simulink model "Simplus_1GFM_2OFF"  (R2022b)
settings: Solver=ode3  StartTime=0.0  StopTime=24  FixedStep=Ts  RelTol=1e-3  EnableMultiTasking=on
InitFcn:
  | Ts = 100e-6;
model workspace (MAT data in the model file):
  Fbase = 50
  Filter_Ind = 0.00435
  Shunt_C = 2.2e-06
  Test_Interval = 3
  Ts = 0.0001
  VDCref = 48
undefined symbols (not defined in the file): DiscIntNeverNeededParam
libraries: rtpi x45, spsabctodq0Lib x2, spsdq0toabcLib x1
settings Model: ModifiedByFormat=The MathWorks Inc.  SimulationMode=external  ExtModeTrigDuration=240000  ExtModeLogAll=off  Creator=The MathWorks, Inc.  LastModifiedBy=The MathWorks Inc.
settings SolverCC: AlgebraicLoopSolver=TrustRegion  PositivePriorityOrder=on  AutoInsertRateTranBlk=on
settings DataIOCC: LimitDataPoints=on  SaveFormat=Array  ReturnWorkspaceOutputs=off
settings OptimizationCC: EnhancedBackFolding=on  PassReuseOutputArgsThreshold=0  LocalBlockOutputs=off  EfficientMapNaN2IntZero=off  MaxStackSize=64  OptimizeBlockOrder=speed  DifferentSizesBufferReuse=on
settings DebuggingCC: UnderspecifiedInitializationDetection=Classic  MergeDetectMultiDrivingBlocksExec=none  SolverPrmCheckMsg=warning  ParameterTunabilityLossMsg=error  UnconnectedInputMsg=warning  UnconnectedOutputMsg=warning  UnconnectedLineMsg=warning  AllowSymbolicDim=off  SFUnexpectedBacktrackingDiag=warning  SFNoUnconditionalDefaultTransitionDiag=warning  SFExecutionAtInitializationDiag=none  SFMachineParentedDataDiag=warning  ArithmeticOperatorsInVariantConditions=warning
settings HardwareCC: ProdBitPerPointer=32  ProdBitPerSizeT=32  ProdBitPerPtrDiffT=32  ProdLargestAtomicInteger=Long  ProdLargestAtomicFloat=Double  ProdWordSize=32  ProdHWDeviceType=ARM Compatible->ARM Cortex  UseEmbeddedCoderFeatures=off
settings ModelReferenceCC: EnableRefExpFcnMdlSchedulingChecks=on  PropagateSignalLabelsOutOfModel=off
settings SFSimCC: SimUseLocalCustomCode=off  SimParseCustomCode=off  MATLABDynamicMemAlloc=off  CustomCodeUndefinedFunction=UseInterfaceOnly
settings RTWCC: Description=Simplus  SystemTargetFile=simplus.tlc  TemplateMakefile=simplex.tmf  RTWUseLocalCustomCode=off  RTWUseSimCustomCode=on  Toolchain=Simplus Xenomai ARM32  BuildConfiguration=Faster Runs
settings CodeAppCC: OperatorAnnotations=on  MangleLength=10  StateflowObjectComments=on
settings STFCustomTargetCC: TargetLangStandard=C99 (ISO)  GenerateFullHeader=off  ConcurrentExecutionCompliant=on  GRTInterface=on  UseToolchainInfoCompliant=on  SystemTargetFile=simplus.tlc
settings GRTTargetCC: GenerateFullHeader=off  ParMdlRefBuildCompliant=off  CompOptLevelCompliant=off  CombineOutputUpdateFcns=off  MatFileLogging=off  CPPClassGenCompliant=off  GRTInterface=on  ExtMode=on  ExtModeMexArgs='192.168.10.109', 0, 17725
settings ConfigComp: CovMetricSettings=dw  CovSaveCumulativeToWorkspaceVar=on  CovSaveSingleToWorkspaceVar=on  CovExternalEMLEnable=off  CovSFcnEnable=off

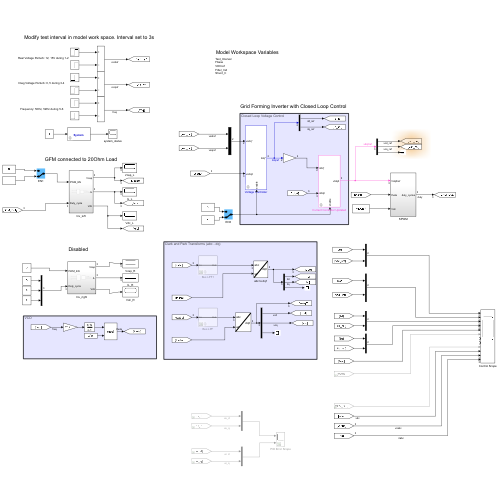
[thumbnail: Simulink's stored preview of the top-level diagram]
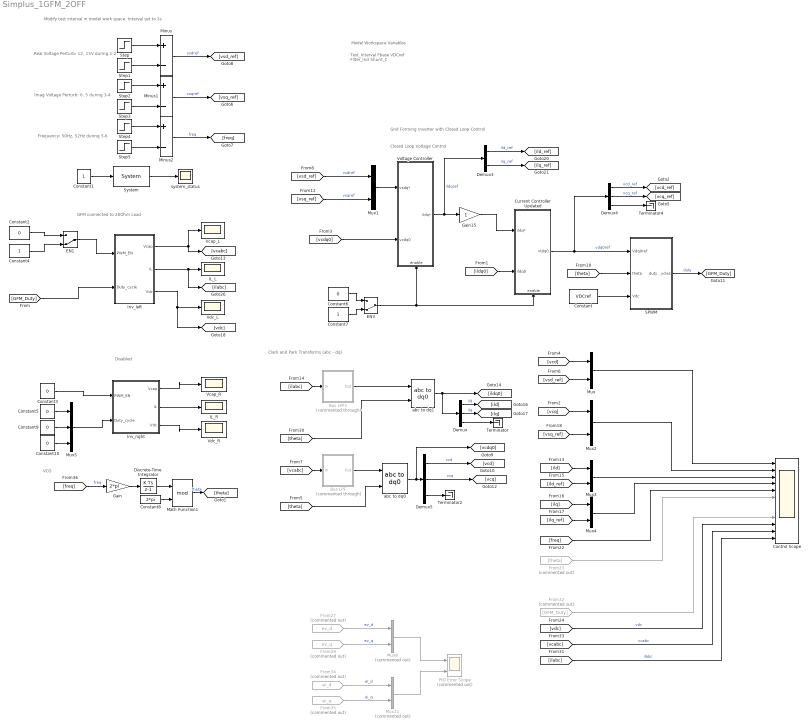
== system Simplus_1GFM_2OFF ==
  note: VCO
  note: Clark and Park Transforms (abc - dq)
  note: Closed Loop Voltage Control
  note: GFM connected to 20Ohm Load
  note: Test_Interval
      | Fbase
      | VDCref
      | Filter_Ind
      | Shunt_C
  note: Model Workspace Variables
  note: Disabled
  note: Grid Forming Inverter with Closed Loop Control
  note: Real Voltage Perturb: 12, 15V during 1-2
  note: Frequency: 50Hz, 52Hz during 5-6
  note: Imag Voltage Perturb: 0, 5 during 3-4
  note: Modify test interval in model work space. Interval set to 3s
  Bus LPF : Subsystem  Commented=through  mask{f_cutoff=1000}
      mask prompts: f_cutoff "Cutoff Frequency (Hz)"
      mask DialogControl Bus_LPF Prompt: Bus LPF
  Bus LPF1 : Subsystem  Commented=through  mask{f_cutoff=1000}
      mask prompts: f_cutoff "Cutoff Frequency (Hz)"
      mask DialogControl Bus_LPF Prompt: Bus LPF
  Constant : Constant  Value=VDCref
  Constant1 : Constant
  Constant{2..3,5..6,9..10} (6 alike) : Constant  Value=0
  Constant4 : Constant
  Constant7 : Constant
  Constant8 : Constant  Value=2*pi
  Control Scope : Scope  NumInputPorts=12
  Current Controller Updated : Subsystem  mask{Id_Proportional=0.61, Id_Integral=240}
      mask prompts: Id_Proportional "Kp"; Id_Integral "Ki"
      settings: PortSchema="{\"entries\":[{\"content\":{\"sides\":[{\"content\":{\"connectorIds\":[\"In1\",\"In2\"]},\"type\":\"ConnectorPlacement.EquallySpacedRectSide\",\"uuid\":\"134caf41-c34b-48d0-a71a-522329c40d8c\"},{\"content\":{\"connectorIds\":[\"Out1\"],\"side\":\"RIGHT\"},\"type\":\"ConnectorPlacement.EquallySpacedRectSide\",\"uuid\":\"de6d8359-09d9-4cb7-8990-bc4b6d48f18d\"},{\"content\":{\"connectorIds\":[],\"side\":\"TOP\"},\"type\":\"ConnectorPlacement.EquallySpacedRectSide\",\"uuid\":\"e2785d07-2ead-4d42-94ac-8025f550e46a\"},{\"content\":{\"connectorIds\":[\"In3\"],\"side\":\"BOTTOM\"},\"type\":\"ConnectorPlacement.EquallySpacedRectSide\",\"uuid\":\"a912a274-012c-4cba-911c-beb79bb7dc91\"}]},\"type\":\"ConnectorPlacement.EquallySpacedConnector\",\"uuid\":\"3c498838-bb9a-4b09-bf48-00f71cabf7b4\"}],\"packageUris\":[\"http://schema.mathworks.com/mf0/Connector/R2020b\"],\"version\":\"1.0\"}"
  Demux : Demux  Outputs=3
  Demux3 : Demux  Outputs=2
  Demux4 : Demux  Outputs=3
  Demux5 : Demux  Outputs=3
  Discrete-Time Integrator : DiscreteIntegrator  SampleTime=Ts  ICPrevOutput=DiscIntNeverNeededParam  ICPrevScaledInput=DiscIntNeverNeededParam
  EN1 : ManualSwitch  CurrentSetting=0
  EN3 : ManualSwitch  CurrentSetting=0
  From23 : From  Commented=on  GotoTag=theta
  From27 : From  Commented=on  GotoTag=ev_d  TagVisibility=global
      settings: CloseFcn=tagdialog Close
  From29 : From  Commented=on  GotoTag=ev_q  TagVisibility=global
      settings: CloseFcn=tagdialog Close
  From32 : From  Commented=on  GotoTag=GFM_Duty
      settings: CloseFcn=tagdialog Close
  From34 : From  Commented=on  GotoTag=ei_d
      settings: CloseFcn=tagdialog Close
  From35 : From  Commented=on  GotoTag=ei_q
      settings: CloseFcn=tagdialog Close
  Gain : Gain  Gain=2*pi
  Gain15 : Gain
  IL_L : Scope
  IL_R : Scope
  Inv_left : Subsystem
  Inv_right : Subsystem
  Math Function1 : Math  Operator=mod  SignedPower=on
  Minus : Sum  Inputs=+-
  Minus1 : Sum  Inputs=+-
  Minus2 : Sum  Inputs=+-
  Mux{,1..4} (5 alike) : Mux  Inputs=2
  Mux11 : Mux  Commented=on  Inputs=2
  Mux5 : Mux  Inputs=3
  Mux8 : Mux  Commented=on  Inputs=2
  PID Error Scope : Scope  Commented=on  NumInputPorts=2
  SPWM : Subsystem
  Step : Step  Time=Test_Interval*1  Before=12  After=15
  Step1 : Step  Time=Test_Interval*2  After=3
  Step2 : Step  Time=Test_Interval*3  After=5
  Step3 : Step  Time=Test_Interval*4  After=5
  Step4 : Step  Time=Test_Interval*5  Before=50  After=52  SampleTime=0
  Step5 : Step  Time=Test_Interval*6  After=2
  System : rtpi/System  Priority=-100  finger_print=015482637925  sync=Synchronous Series  div=4  estop=NONE
      settings: SourceProductName=Simplus Real-Time
  Terminator : Terminator
  Terminator2 : Terminator
  Terminator4 : Terminator
  Vcap_L : Scope
  Vcap_R : Scope
  Vdc_L : Scope
  Vdc_R : Scope
  Voltage Controller : Subsystem  mask{Id_Proportional=0.028, Id_Integral=8.685}
      mask prompts: Id_Proportional "Kp"; Id_Integral "Ki"
      settings: PortSchema="{\"entries\":[{\"content\":{\"sides\":[{\"content\":{\"connectorIds\":[\"In1\",\"In2\"]},\"type\":\"ConnectorPlacement.EquallySpacedRectSide\",\"uuid\":\"134caf41-c34b-48d0-a71a-522329c40d8c\"},{\"content\":{\"connectorIds\":[\"Out1\"],\"side\":\"RIGHT\"},\"type\":\"ConnectorPlacement.EquallySpacedRectSide\",\"uuid\":\"de6d8359-09d9-4cb7-8990-bc4b6d48f18d\"},{\"content\":{\"connectorIds\":[],\"side\":\"TOP\"},\"type\":\"ConnectorPlacement.EquallySpacedRectSide\",\"uuid\":\"e2785d07-2ead-4d42-94ac-8025f550e46a\"},{\"content\":{\"connectorIds\":[\"In3\"],\"side\":\"BOTTOM\"},\"type\":\"ConnectorPlacement.EquallySpacedRectSide\",\"uuid\":\"a912a274-012c-4cba-911c-beb79bb7dc91\"}]},\"type\":\"ConnectorPlacement.EquallySpacedConnector\",\"uuid\":\"3c498838-bb9a-4b09-bf48-00f71cabf7b4\"}],\"packageUris\":[\"http://schema.mathworks.com/mf0/Connector/R2020b\"],\"version\":\"1.0\"}"
  abc to dq0 : spsabctodq0Lib/abc to dq0  Alignment=90 degrees behind phase A axis
  abc to dq1 : spsabctodq0Lib/abc to dq0  Alignment=90 degrees behind phase A axis
  system_status : Scope
  wires:
  System/1 -> system_status/1
  Constant1/1 -> System/1
  Constant2/1 -> EN1/1
  Constant4/1 -> EN1/2
  EN1/1 -> Inv_left/1(PWM_EN)
  Inv_left/3(Vdc) -> [vdc], Vdc_L/1
  Inv_right/1(Vcap) -> Vcap_R/1
  Constant3/1 -> Inv_right/1(PWM_EN)
  Inv_right/2(IL) -> IL_R/1
  Demux4/2 -> [vcq_ref]  "vcq_ref"
  Demux/2 -> [ilq]  "ilq"
  Demux4/3 -> Terminator4/1
  Demux3/2 -> [ilq_ref]  "ilq_ref"
  Demux/3 -> Terminator/1
  Voltage Controller/1(ildq*) -> Gain15/1, Demux3/1  "ildqref"
  Current Controller Updated/1(vtdq0) -> Demux4/1, SPWM/1(Vdq0ref)  "vdq0ref"
  [theta] -> SPWM/2(theta)
  [ilabc] -> Bus LPF1/1(In)
  SPWM/1(duty_cycles) -> [GFM_Duty]  "duty"
  Demux/1 -> [ild]  "ild"
  EN3/1 -> Current Controller Updated/3(enable), Voltage Controller/3(enable)
  Demux3/1 -> [ild_ref]  "ild_ref"
  Demux4/1 -> [vcd_ref]  "vcd_ref"
  Constant/1 -> SPWM/3(Vdc)
  Gain15/1 -> Current Controller Updated/1(ildq*)
  Constant6/1 -> EN3/1
  Constant7/1 -> EN3/2
  [vcd] -> Mux/1
  [vcq] -> Mux2/1
  [ild] -> Mux3/1
  [ild_ref] -> Mux3/2
  [ilq] -> Mux4/1
  [ilq_ref] -> Mux4/2
  Mux/1 -> Control Scope/1
  Mux2/1 -> Control Scope/2
  Mux3/1 -> Control Scope/3
  Mux4/1 -> Control Scope/4
  From23/1 -> Control Scope/6
  Gain/1 -> Discrete-Time Integrator/1
  Discrete-Time Integrator/1 -> Math Function1/1
  Constant8/1 -> Math Function1/2
  [freq] -> Gain/1  "freq"
  Math Function1/1 -> [theta]  "theta"
  abc to dq0/1 -> [vcdq0], Demux5/1
  Demux5/1 -> [vcd]  "vcd"
  Demux5/3 -> Terminator2/1
  Demux5/2 -> [vcq]  "vcq"
  [vcabc] -> Bus LPF/1(In)
  [theta] -> abc to dq1/2
  abc to dq1/1 -> [ildq0], Demux/1
  [ilabc] -> Control Scope/12  "ilabc"
  [vcabc] -> Control Scope/11  "vcabc"
  From32/1 -> Control Scope/9
  [vcdq0] -> Voltage Controller/2(vcdq0)
  Bus LPF1/1(Out) -> abc to dq1/1
  [freq] -> Control Scope/5
  Inv_left/1(Vcap) -> Vcap_L/1, [vcabc]
  Inv_left/2(IL) -> [ilabc], IL_L/1
  [GFM_Duty] -> Inv_left/2(Duty_cycle)
  [vsq_ref] -> Mux1/2  "vsqref"
  Mux1/1 -> Voltage Controller/1(vsdq*)
  [vsd_ref] -> Mux1/1  "vsdref"
  Constant5/1 -> Mux5/1
  Constant9/1 -> Mux5/2
  Constant10/1 -> Mux5/3
  Mux5/1 -> Inv_right/2(Duty_cycle)
  [theta] -> abc to dq0/2
  [vsq_ref] -> Mux2/2
  [vsd_ref] -> Mux/2
  [vdc] -> Control Scope/10  "vdc"
  Inv_right/3(Vdc) -> Vdc_R/1
  Mux8/1 -> PID Error Scope/1
  From27/1 -> Mux8/1  "ev_d"
  From29/1 -> Mux8/2  "ev_q"
  From35/1 -> Mux11/2  "ei_q"
  Mux11/1 -> PID Error Scope/2
  From34/1 -> Mux11/1  "ei_d"
  Bus LPF/1(Out) -> abc to dq0/1
  [ildq0] -> Current Controller Updated/2(ildq0)
  Minus1/1 -> [vsq_ref]  "vsqref"
  Step3/1 -> Minus1/2
  Step5/1 -> Minus2/2
  Minus2/1 -> [freq]  "freq"
  Step4/1 -> Minus2/1
  Step2/1 -> Minus1/1
  Step/1 -> Minus/1
  Minus/1 -> [vsd_ref]  "vsdref"
  Step1/1 -> Minus/2

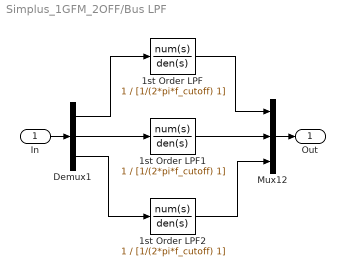
== system Simplus_1GFM_2OFF/Bus LPF ==
  In : Inport
  1st Order LPF : TransferFcn  Numerator=1  Denominator=[1/(2*pi*f_cutoff) 1]
  1st Order LPF1 : TransferFcn  Numerator=1  Denominator=[1/(2*pi*f_cutoff) 1]
  1st Order LPF2 : TransferFcn  Numerator=1  Denominator=[1/(2*pi*f_cutoff) 1]
  Demux1 : Demux  Outputs=3
  Mux12 : Mux  Inputs=3
  Out : Outport
  wires:
  Demux1/3 -> 1st Order LPF2/1
  Mux12/1 -> Out/1
  1st Order LPF/1 -> Mux12/1
  Demux1/1 -> 1st Order LPF/1
  Demux1/2 -> 1st Order LPF1/1
  1st Order LPF2/1 -> Mux12/3
  In/1 -> Demux1/1
  1st Order LPF1/1 -> Mux12/2

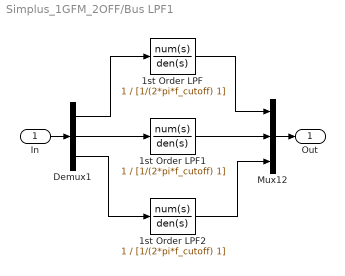
== system Simplus_1GFM_2OFF/Bus LPF1 ==
  In : Inport
  1st Order LPF : TransferFcn  Numerator=1  Denominator=[1/(2*pi*f_cutoff) 1]
  1st Order LPF1 : TransferFcn  Numerator=1  Denominator=[1/(2*pi*f_cutoff) 1]
  1st Order LPF2 : TransferFcn  Numerator=1  Denominator=[1/(2*pi*f_cutoff) 1]
  Demux1 : Demux  Outputs=3
  Mux12 : Mux  Inputs=3
  Out : Outport
  wires:
  Demux1/3 -> 1st Order LPF2/1
  Mux12/1 -> Out/1
  1st Order LPF/1 -> Mux12/1
  Demux1/1 -> 1st Order LPF/1
  Demux1/2 -> 1st Order LPF1/1
  1st Order LPF2/1 -> Mux12/3
  In/1 -> Demux1/1
  1st Order LPF1/1 -> Mux12/2

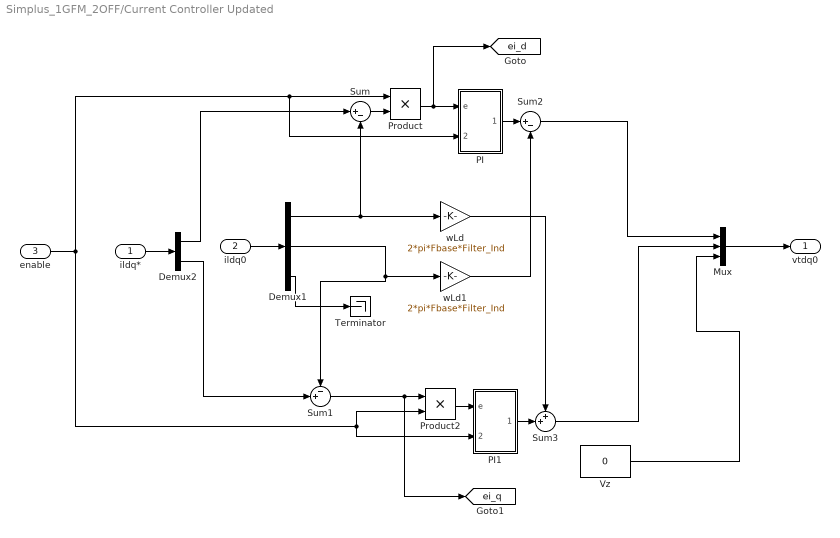
== system Simplus_1GFM_2OFF/Current Controller Updated ==
  ildq* : Inport
  ildq0 : Inport  Port=2
  enable : Inport  Port=3
  Demux1 : Demux  Outputs=3
  Demux2 : Demux  Outputs=2
  Mux : Mux  Inputs=3
  PI : Subsystem
  PI1 : Subsystem
  Product : Product  RndMeth=Zero
  Product2 : Product  RndMeth=Zero
  Sum : Sum  Inputs=|+-
  Sum1 : Sum  Inputs=-+|
  Sum2 : Sum  Inputs=|+-
  Sum3 : Sum  Inputs=++|
  Terminator : Terminator
  Vz : Constant  Value=0
  wLd : Gain  Gain=2*pi*Fbase*Filter_Ind
  wLd1 : Gain  Gain=2*pi*Fbase*Filter_Ind
  vtdq0 : Outport
  tag scope: ei_d=global, ei_q=global
  wires:
  Sum2/1 -> Mux/1
  Sum3/1 -> Mux/2
  ildq0/1 -> Demux1/1
  Mux/1 -> vtdq0/1
  Demux1/3 -> Terminator/1
  ildq*/1 -> Demux2/1
  Demux2/1 -> Sum/1
  Demux2/2 -> Sum1/2
  PI/1(Out) -> Sum2/1
  wLd/1 -> Sum3/1
  wLd1/1 -> Sum2/2
  PI1/1(Out) -> Sum3/2
  Demux1/2 -> Sum1/1, wLd1/1
  Demux1/1 -> wLd/1, Sum/2
  Product2/1 -> PI1/1(e)
  Sum/1 -> Product/2
  enable/1 -> Product/1, PI/2(RST), PI1/2(RST), Product2/2
  Vz/1 -> Mux/3
  Sum1/1 -> [ei_q], Product2/1
  Product/1 -> [ei_d], PI/1(e)

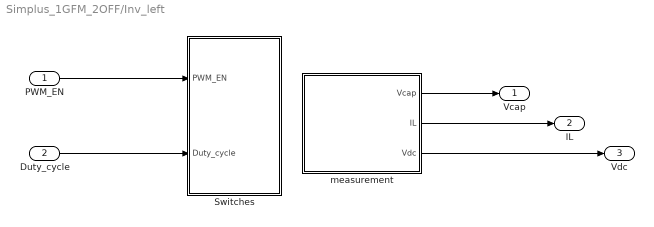
== system Simplus_1GFM_2OFF/Inv_left ==
  PWM_EN : Inport
  Duty_cycle : Inport  Port=2
  Switches : Subsystem
  measurement : Subsystem
  Vcap : Outport
  IL : Outport  Port=2
  Vdc : Outport  Port=3
  wires:
  Duty_cycle/1 -> Switches/2(Duty_cycle)
  PWM_EN/1 -> Switches/1(PWM_EN)
  measurement/3(Vdc) -> Vdc/1
  measurement/2(IL) -> IL/1
  measurement/1(Vcap) -> Vcap/1

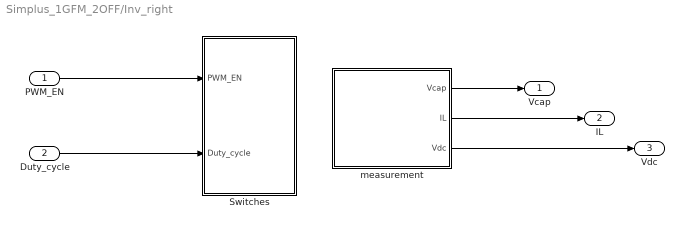
== system Simplus_1GFM_2OFF/Inv_right ==
  PWM_EN : Inport
  Duty_cycle : Inport  Port=2
  Switches : Subsystem
  measurement : Subsystem
  Vcap : Outport
  IL : Outport  Port=2
  Vdc : Outport  Port=3
  wires:
  measurement/1(Vcap) -> Vcap/1
  measurement/2(IL) -> IL/1
  measurement/3(Vdc) -> Vdc/1
  PWM_EN/1 -> Switches/1(PWM_EN)
  Duty_cycle/1 -> Switches/2(Duty_cycle)

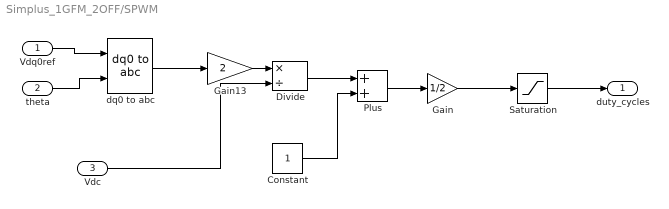
== system Simplus_1GFM_2OFF/SPWM ==
  Vdq0ref : Inport
  theta : Inport  Port=2
  Vdc : Inport  Port=3
  Constant : Constant
  Divide : Product  Inputs=*/
  Gain : Gain  Gain=1/2
  Gain13 : Gain  Gain=2
  Plus : Sum
  Saturation : Saturate  UpperLimit=0.9  LowerLimit=0.1
  dq0 to abc : spsdq0toabcLib/dq0 to abc  Alignment=90 degrees behind phase A axis
  duty_cycles : Outport
  wires:
  Vdq0ref/1 -> dq0 to abc/1
  Gain/1 -> Saturation/1
  theta/1 -> dq0 to abc/2
  Constant/1 -> Plus/2
  Plus/1 -> Gain/1
  Saturation/1 -> duty_cycles/1
  dq0 to abc/1 -> Gain13/1
  Gain13/1 -> Divide/1
  Vdc/1 -> Divide/2
  Divide/1 -> Plus/1

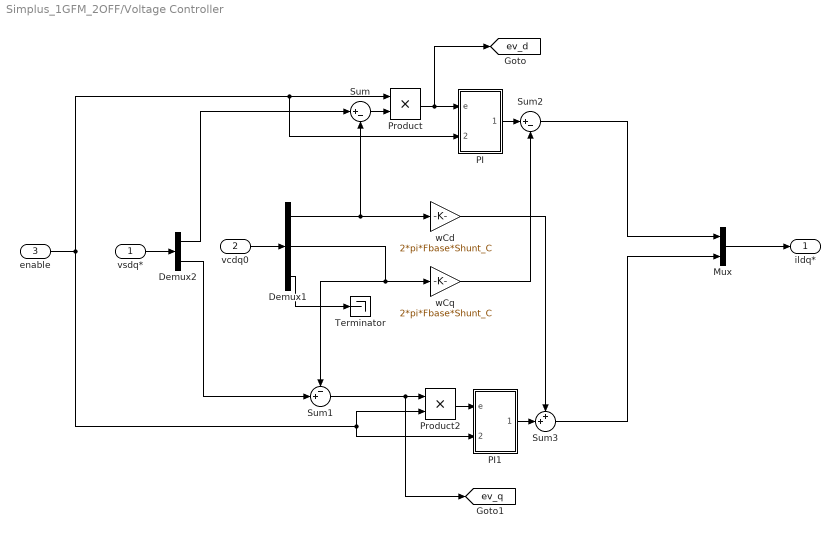
== system Simplus_1GFM_2OFF/Voltage Controller ==
  vsdq* : Inport
  vcdq0 : Inport  Port=2
  enable : Inport  Port=3
  Demux1 : Demux  Outputs=3
  Demux2 : Demux  Outputs=2
  Mux : Mux  Inputs=2
  PI : Subsystem
  PI1 : Subsystem
  Product : Product  RndMeth=Zero
  Product2 : Product  RndMeth=Zero
  Sum : Sum  Inputs=|+-
  Sum1 : Sum  Inputs=-+|
  Sum2 : Sum  Inputs=|+-
  Sum3 : Sum  Inputs=++|
  Terminator : Terminator
  wCd : Gain  Gain=2*pi*Fbase*Shunt_C
  wCq : Gain  Gain=2*pi*Fbase*Shunt_C
  ildq* : Outport
  tag scope: ev_d=global, ev_q=global
  wires:
  Sum2/1 -> Mux/1
  Sum3/1 -> Mux/2
  vcdq0/1 -> Demux1/1
  Mux/1 -> ildq*/1
  Demux1/3 -> Terminator/1
  vsdq*/1 -> Demux2/1
  Demux2/1 -> Sum/1
  Demux2/2 -> Sum1/2
  Product/1 -> [ev_d], PI/1(e)
  Sum1/1 -> [ev_q], Product2/1
  PI/1(Out) -> Sum2/1
  wCd/1 -> Sum3/1
  wCq/1 -> Sum2/2
  PI1/1(Out) -> Sum3/2
  Demux1/2 -> Sum1/1, wCq/1
  Demux1/1 -> wCd/1, Sum/2
  Product2/1 -> PI1/1(e)
  Sum/1 -> Product/2
  enable/1 -> Product/1, PI/2(RST), PI1/2(RST), Product2/2

== system Simplus_1GFM_2OFF/Current Controller Updated/PI ==
  e : Inport
  RST : Inport  Port=2
  Discrete-Time Integrator : DiscreteIntegrator  gainval=1  ExternalReset=either  SampleTime=Ts  LimitOutput=on  UpperSaturationLimit=20000  LowerSaturationLimit=-20000  ICPrevOutput=DiscIntNeverNeededParam  ICPrevScaledInput=DiscIntNeverNeededParam
  Ki : Gain  Gain=Id_Integral  SaturateOnIntegerOverflow=on  OutDataTypeStr=Inherit: Same as input  ParamDataTypeStr=Inherit: Same as input
  Kp : Gain  Gain=Id_Proportional  SaturateOnIntegerOverflow=on  OutDataTypeStr=Inherit: Same as input  ParamDataTypeStr=Inherit: Same as input
  Sum4 : Sum  SaturateOnIntegerOverflow=on
  Out : Outport
  wires:
  Ki/1 -> Discrete-Time Integrator/1
  Kp/1 -> Sum4/1
  e/1 -> Ki/1, Kp/1
  Discrete-Time Integrator/1 -> Sum4/2
  Sum4/1 -> Out/1
  RST/1 -> Discrete-Time Integrator/2

== system Simplus_1GFM_2OFF/Current Controller Updated/PI1 ==
  e : Inport
  RST : Inport  Port=2
  Discrete-Time Integrator : DiscreteIntegrator  gainval=1  ExternalReset=either  SampleTime=Ts  LimitOutput=on  UpperSaturationLimit=20000  LowerSaturationLimit=-20000  ICPrevOutput=DiscIntNeverNeededParam  ICPrevScaledInput=DiscIntNeverNeededParam
  Ki : Gain  Gain=Id_Integral  SaturateOnIntegerOverflow=on  OutDataTypeStr=Inherit: Same as input  ParamDataTypeStr=Inherit: Same as input
  Kp : Gain  Gain=Id_Proportional  SaturateOnIntegerOverflow=on  OutDataTypeStr=Inherit: Same as input  ParamDataTypeStr=Inherit: Same as input
  Sum4 : Sum  SaturateOnIntegerOverflow=on
  Out : Outport
  wires:
  Ki/1 -> Discrete-Time Integrator/1
  Kp/1 -> Sum4/1
  e/1 -> Ki/1, Kp/1
  Discrete-Time Integrator/1 -> Sum4/2
  Sum4/1 -> Out/1
  RST/1 -> Discrete-Time Integrator/2

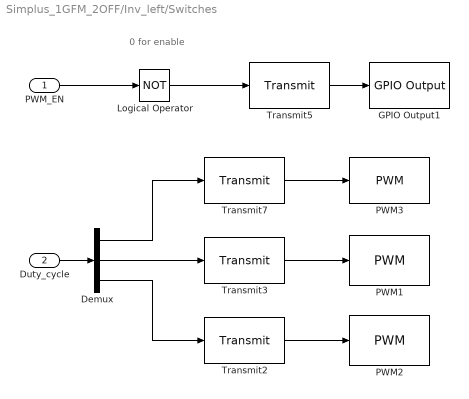
== system Simplus_1GFM_2OFF/Inv_left/Switches ==
  note: 0 for enable
  PWM_EN : Inport
  Duty_cycle : Inport  Port=2
  Demux : Demux  Outputs=3
  GPIO Output1 : rtpi/GPIO Output  finger_print=115482637925  blk_num=1  gpio_num=1  gpio1=18  od1=off  gpio2=0  od2=off  gpio3=0  od3=off  gpio4=0  od4=off  gpio5=0  od5=off  gpio6=0  od6=off  gpio7=0  od7=off  gpio8=0  od8=off  gpio9=0  od9=off  gpio10=0  od10=off  gpio11=0  od11=off  gpio12=0  od12=off  gpio13=0  od13=off  gpio14=0  od14=off  gpio15=0  od15=off  gpio16=0  od16=off  dir=1
      settings: SourceProductName=Simplus Real-Time
  Logical Operator : Logic  Operator=NOT  AllPortsSameDT=off  OutDataTypeStr=boolean
  PWM1 : rtpi/PWM  finger_print=115482637925  blk_num=1  pwmx=5  sync=on  mode=Normal  input=Duty Cycle  data_type=float  trigger_a=Zero  trigger_b=Zero  clock=1  tdead=2  period=10000  duty=0.5  phase=0.0
      settings: SourceProductName=Simplus Real-Time
  PWM2 : rtpi/PWM  finger_print=115482637925  blk_num=2  pwmx=6  sync=on  mode=Normal  input=Duty Cycle  data_type=float  trigger_a=Zero  trigger_b=Zero  clock=1  tdead=2  period=10000  duty=0.5  phase=0.0
      settings: SourceProductName=Simplus Real-Time
  PWM3 : rtpi/PWM  finger_print=115482637925  blk_num=3  pwmx=4  sync=on  mode=Normal  input=Duty Cycle  data_type=float  trigger_a=Zero  trigger_b=Zero  clock=1  tdead=2  period=10000  duty=0.5  phase=0.0
      settings: SourceProductName=Simplus Real-Time
  Transmit2 : rtpi/Transmit  Priority=10  finger_print=115482637925  blk_num=1  data_type=4  conv_type=single
      settings: SourceProductName=Simplus Real-Time
  Transmit3 : rtpi/Transmit  Priority=10  finger_print=115482637925  blk_num=2  data_type=4  conv_type=single
      settings: SourceProductName=Simplus Real-Time
  Transmit5 : rtpi/Transmit  finger_print=115482637925  blk_num=3  data_type=2  conv_type=uint16
      settings: SourceProductName=Simplus Real-Time
  Transmit7 : rtpi/Transmit  Priority=10  finger_print=115482637925  blk_num=4  data_type=4  conv_type=single
      settings: SourceProductName=Simplus Real-Time
  wires:
  Transmit2/1 -> PWM2/1
  Transmit3/1 -> PWM1/1
  Transmit7/1 -> PWM3/1
  Duty_cycle/1 -> Demux/1
  Demux/2 -> Transmit3/1
  Demux/1 -> Transmit7/1
  Demux/3 -> Transmit2/1
  Transmit5/1 -> GPIO Output1/1
  Logical Operator/1 -> Transmit5/1
  PWM_EN/1 -> Logical Operator/1

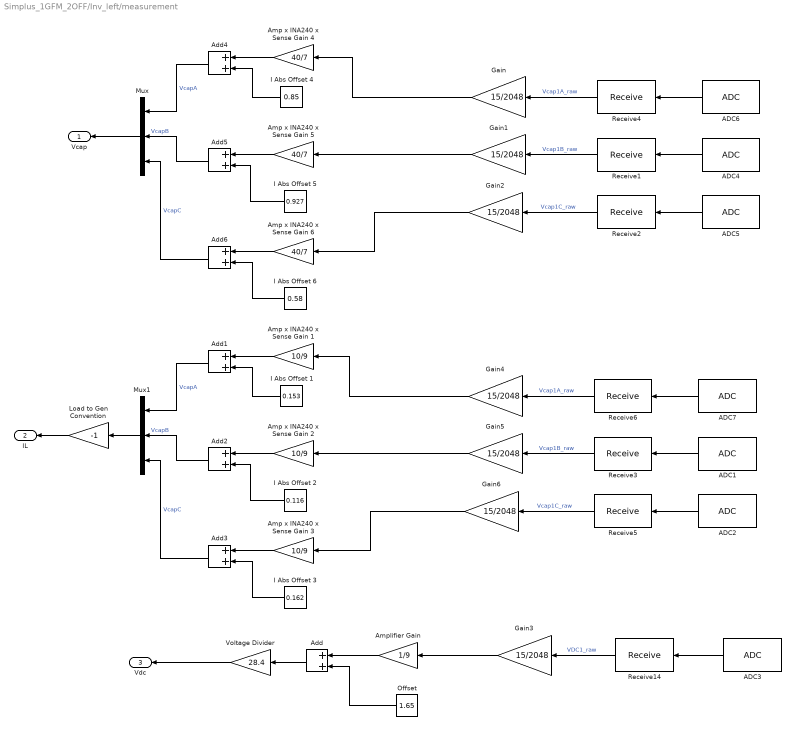
== system Simplus_1GFM_2OFF/Inv_left/measurement ==
  ADC1 : rtpi/ADC  finger_print=115482637925  blk_num=1  adcx=D  prior=2  pin=D2  trigger=PWM4A  data_type=int16  gain=1  rsrc=100  offset=AC  protect=Enabled  max=2000  min=-2000
      settings: SourceProductName=Simplus Real-Time
  ADC2 : rtpi/ADC  finger_print=115482637925  blk_num=2  adcx=D  prior=3  pin=D3  trigger=PWM4A  data_type=int16  gain=1  rsrc=100  offset=AC  protect=Enabled  max=2000  min=-2000
      settings: SourceProductName=Simplus Real-Time
  ADC3 : rtpi/ADC  finger_print=115482637925  blk_num=3  adcx=D  prior=4  pin=D4  trigger=PWM4A  data_type=int16  gain=1  rsrc=100  offset=AC  protect=Enabled  max=1500  min=-2048
      settings: SourceProductName=Simplus Real-Time
  ADC4 : rtpi/ADC  finger_print=115482637925  blk_num=4  adcx=C  prior=2  pin=C2  trigger=PWM4A  data_type=int16  gain=1  rsrc=100  offset=AC  protect=Enabled  max=2000  min=-2000
      settings: SourceProductName=Simplus Real-Time
  ADC5 : rtpi/ADC  finger_print=115482637925  blk_num=5  adcx=C  prior=3  pin=C3  trigger=PWM4A  data_type=int16  gain=1  rsrc=100  offset=AC  protect=Enabled  max=2000  min=-2000
      settings: SourceProductName=Simplus Real-Time
  ADC6 : rtpi/ADC  finger_print=115482637925  blk_num=6  adcx=C  prior=1  pin=C1  trigger=PWM4A  data_type=int16  gain=1  rsrc=100  offset=AC  protect=Enabled  max=2000  min=-2000
      settings: SourceProductName=Simplus Real-Time
  ADC7 : rtpi/ADC  finger_print=115482637925  blk_num=7  adcx=D  prior=1  pin=D1  trigger=PWM4A  data_type=int16  gain=1  rsrc=100  offset=AC  protect=Enabled  max=2000  min=-2000
      settings: SourceProductName=Simplus Real-Time
  Add{,1..6} (7 alike) : Sum
  Amp x INA240 x Sense Gain 1 : Gain  Gain=10/9
  Amp x INA240 x Sense Gain 2 : Gain  Gain=10/9
  Amp x INA240 x Sense Gain 3 : Gain  Gain=10/9
  Amp x INA240 x Sense Gain 4 : Gain  Gain=40/7
  Amp x INA240 x Sense Gain 5 : Gain  Gain=40/7
  Amp x INA240 x Sense Gain 6 : Gain  Gain=40/7
  Amplifier Gain : Gain  Gain=1/9
  Gain{,1..6} (7 alike) : Gain  Gain=15/2048
  I Abs Offset 1 : Constant  Value=0.153
  I Abs Offset 2 : Constant  Value=0.116
  I Abs Offset 3 : Constant  Value=0.162
  I Abs Offset 4 : Constant  Value=0.85
  I Abs Offset 5 : Constant  Value=0.927
  I Abs Offset 6 : Constant  Value=0.58
  Load to Gen Convention : Gain  Gain=-1
  Mux : Mux  Inputs=3
  Mux1 : Mux  Inputs=3
  Offset : Constant  Value=1.65
  Receive1 : rtpi/Receive  Priority=12  finger_print=115482637925  blk_num=1  data_type=2
      settings: SourceProductName=Simplus Real-Time
  Receive14 : rtpi/Receive  Priority=12  finger_print=115482637925  blk_num=2  data_type=2
      settings: SourceProductName=Simplus Real-Time
  Receive2 : rtpi/Receive  Priority=12  finger_print=115482637925  blk_num=3  data_type=2
      settings: SourceProductName=Simplus Real-Time
  Receive3 : rtpi/Receive  Priority=12  finger_print=115482637925  blk_num=4  data_type=2
      settings: SourceProductName=Simplus Real-Time
  Receive4 : rtpi/Receive  Priority=12  finger_print=115482637925  blk_num=5  data_type=2
      settings: SourceProductName=Simplus Real-Time
  Receive5 : rtpi/Receive  Priority=12  finger_print=115482637925  blk_num=6  data_type=2
      settings: SourceProductName=Simplus Real-Time
  Receive6 : rtpi/Receive  Priority=12  finger_print=115482637925  blk_num=7  data_type=2
      settings: SourceProductName=Simplus Real-Time
  Voltage Divider : Gain  Gain=28.4
  Vcap : Outport
  IL : Outport  Port=2
  Vdc : Outport  Port=3
  wires:
  ADC6/1 -> Receive4/1
  Receive4/1 -> Gain/1  "Vcap1A_raw"
  Amp x INA240 x Sense Gain 6/1 -> Add6/1
  I Abs Offset 6/1 -> Add6/2
  I Abs Offset 4/1 -> Add4/2
  Amp x INA240 x Sense Gain 4/1 -> Add4/1
  ADC5/1 -> Receive2/1
  Amp x INA240 x Sense Gain 5/1 -> Add5/1
  Receive1/1 -> Gain1/1  "Vcap1B_raw"
  I Abs Offset 5/1 -> Add5/2
  Receive2/1 -> Gain2/1  "Vcap1C_raw"
  ADC4/1 -> Receive1/1
  Amp x INA240 x Sense Gain 3/1 -> Add3/1
  Amp x INA240 x Sense Gain 1/1 -> Add1/1
  I Abs Offset 1/1 -> Add1/2
  Amp x INA240 x Sense Gain 2/1 -> Add2/1
  I Abs Offset 2/1 -> Add2/2
  I Abs Offset 3/1 -> Add3/2
  Receive14/1 -> Gain3/1  "VDC1_raw"
  ADC3/1 -> Receive14/1
  Add/1 -> Voltage Divider/1
  Amplifier Gain/1 -> Add/1
  Offset/1 -> Add/2
  Voltage Divider/1 -> Vdc/1
  Gain/1 -> Amp x INA240 x Sense Gain 4/1
  Gain1/1 -> Amp x INA240 x Sense Gain 5/1
  Gain2/1 -> Amp x INA240 x Sense Gain 6/1
  Gain3/1 -> Amplifier Gain/1
  Add4/1 -> Mux/1  "VcapA"
  Add5/1 -> Mux/2  "VcapB"
  Add6/1 -> Mux/3  "VcapC"
  Mux/1 -> Vcap/1
  ADC7/1 -> Receive6/1
  Gain4/1 -> Amp x INA240 x Sense Gain 1/1
  Gain5/1 -> Amp x INA240 x Sense Gain 2/1
  ADC1/1 -> Receive3/1
  ADC2/1 -> Receive5/1
  Receive3/1 -> Gain5/1  "Vcap1B_raw"
  Receive5/1 -> Gain6/1  "Vcap1C_raw"
  Gain6/1 -> Amp x INA240 x Sense Gain 3/1
  Receive6/1 -> Gain4/1  "Vcap1A_raw"
  Add3/1 -> Mux1/3  "VcapC"
  Mux1/1 -> Load to Gen Convention/1
  Add1/1 -> Mux1/1  "VcapA"
  Add2/1 -> Mux1/2  "VcapB"
  Load to Gen Convention/1 -> IL/1

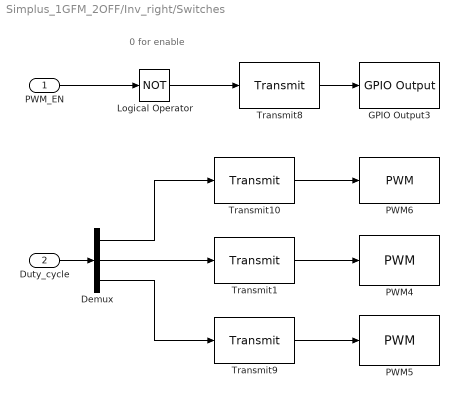
== system Simplus_1GFM_2OFF/Inv_right/Switches ==
  note: 0 for enable
  PWM_EN : Inport
  Duty_cycle : Inport  Port=2
  Demux : Demux  Outputs=3
  GPIO Output3 : rtpi/GPIO Output  finger_print=115482637925  blk_num=2  gpio_num=1  gpio1=24  od1=off  gpio2=0  od2=off  gpio3=0  od3=off  gpio4=0  od4=off  gpio5=0  od5=off  gpio6=0  od6=off  gpio7=0  od7=off  gpio8=0  od8=off  gpio9=0  od9=off  gpio10=0  od10=off  gpio11=0  od11=off  gpio12=0  od12=off  gpio13=0  od13=off  gpio14=0  od14=off  gpio15=0  od15=off  gpio16=0  od16=off  dir=1
      settings: SourceProductName=Simplus Real-Time
  Logical Operator : Logic  Operator=NOT  AllPortsSameDT=off  OutDataTypeStr=boolean
  PWM4 : rtpi/PWM  finger_print=115482637925  blk_num=4  pwmx=2  sync=on  mode=Normal  input=Duty Cycle  data_type=float  trigger_a=Zero  trigger_b=Zero  clock=1  tdead=2  period=10000  duty=0.5  phase=0.0
      settings: SourceProductName=Simplus Real-Time
  PWM5 : rtpi/PWM  finger_print=115482637925  blk_num=5  pwmx=3  sync=on  mode=Normal  input=Duty Cycle  data_type=float  trigger_a=Zero  trigger_b=Zero  clock=1  tdead=2  period=10000  duty=0.5  phase=0.0
      settings: SourceProductName=Simplus Real-Time
  PWM6 : rtpi/PWM  finger_print=115482637925  blk_num=6  pwmx=1  sync=on  mode=Normal  input=Duty Cycle  data_type=float  trigger_a=Zero  trigger_b=Zero  clock=1  tdead=2  period=10000  duty=0.5  phase=0.0
      settings: SourceProductName=Simplus Real-Time
  Transmit1 : rtpi/Transmit  Priority=10  finger_print=115482637925  blk_num=5  data_type=4  conv_type=single
      settings: SourceProductName=Simplus Real-Time
  Transmit10 : rtpi/Transmit  Priority=10  finger_print=115482637925  blk_num=6  data_type=4  conv_type=single
      settings: SourceProductName=Simplus Real-Time
  Transmit8 : rtpi/Transmit  finger_print=115482637925  blk_num=7  data_type=2  conv_type=uint16
      settings: SourceProductName=Simplus Real-Time
  Transmit9 : rtpi/Transmit  Priority=10  finger_print=115482637925  blk_num=8  data_type=4  conv_type=single
      settings: SourceProductName=Simplus Real-Time
  wires:
  Duty_cycle/1 -> Demux/1
  PWM_EN/1 -> Logical Operator/1
  Demux/3 -> Transmit9/1
  Demux/1 -> Transmit10/1
  Demux/2 -> Transmit1/1
  Transmit9/1 -> PWM5/1
  Transmit1/1 -> PWM4/1
  Transmit10/1 -> PWM6/1
  Transmit8/1 -> GPIO Output3/1
  Logical Operator/1 -> Transmit8/1

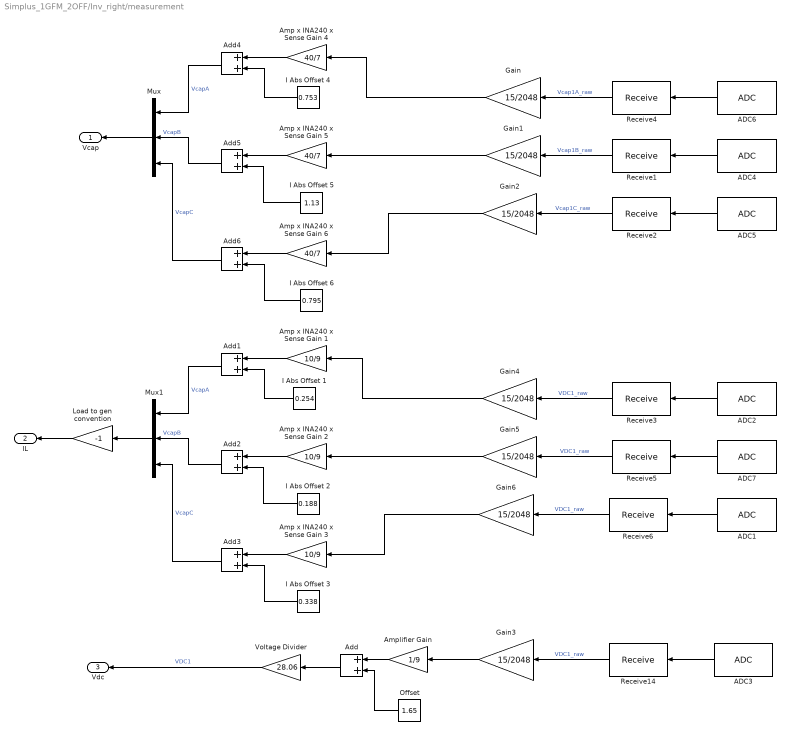
== system Simplus_1GFM_2OFF/Inv_right/measurement ==
  ADC1 : rtpi/ADC  finger_print=115482637925  blk_num=8  adcx=A  prior=1  pin=A1  trigger=PWM1A  data_type=int16  gain=1  rsrc=100  offset=AC  protect=Enabled  max=1500  min=-1500
      settings: SourceProductName=Simplus Real-Time
  ADC2 : rtpi/ADC  finger_print=115482637925  blk_num=9  adcx=A  prior=2  pin=A2  trigger=PWM1A  data_type=int16  gain=1  rsrc=100  offset=AC  protect=Enabled  max=1500  min=-1500
      settings: SourceProductName=Simplus Real-Time
  ADC3 : rtpi/ADC  finger_print=115482637925  blk_num=10  adcx=A  prior=4  pin=A4  trigger=PWM1A  data_type=int16  gain=1  rsrc=100  offset=AC  protect=Enabled  max=1500  min=-2048
      settings: SourceProductName=Simplus Real-Time
  ADC4 : rtpi/ADC  finger_print=115482637925  blk_num=11  adcx=B  prior=2  pin=B3  trigger=PWM1A  data_type=int16  gain=1  rsrc=100  offset=AC  protect=Enabled  max=1500  min=-1500
      settings: SourceProductName=Simplus Real-Time
  ADC5 : rtpi/ADC  finger_print=115482637925  blk_num=12  adcx=B  prior=3  pin=B4  trigger=PWM1A  data_type=int16  gain=1  rsrc=100  offset=AC  protect=Enabled  max=1500  min=-1500
      settings: SourceProductName=Simplus Real-Time
  ADC6 : rtpi/ADC  finger_print=115482637925  blk_num=13  adcx=B  prior=1  pin=B2  trigger=PWM1A  data_type=int16  gain=1  rsrc=100  offset=AC  protect=Enabled  max=1500  min=-1500
      settings: SourceProductName=Simplus Real-Time
  ADC7 : rtpi/ADC  finger_print=115482637925  blk_num=14  adcx=A  prior=3  pin=A3  trigger=PWM1A  data_type=int16  gain=1  rsrc=100  offset=AC  protect=Enabled  max=1500  min=-1500
      settings: SourceProductName=Simplus Real-Time
  Add{,1..6} (7 alike) : Sum
  Amp x INA240 x Sense Gain 1 : Gain  Gain=10/9
  Amp x INA240 x Sense Gain 2 : Gain  Gain=10/9
  Amp x INA240 x Sense Gain 3 : Gain  Gain=10/9
  Amp x INA240 x Sense Gain 4 : Gain  Gain=40/7
  Amp x INA240 x Sense Gain 5 : Gain  Gain=40/7
  Amp x INA240 x Sense Gain 6 : Gain  Gain=40/7
  Amplifier Gain : Gain  Gain=1/9
  Gain{,1..6} (7 alike) : Gain  Gain=15/2048
  I Abs Offset 1 : Constant  Value=0.254
  I Abs Offset 2 : Constant  Value=0.188
  I Abs Offset 3 : Constant  Value=0.338
  I Abs Offset 4 : Constant  Value=0.753
  I Abs Offset 5 : Constant  Value=1.13
  I Abs Offset 6 : Constant  Value=0.795
  Load to gen convention : Gain  Gain=-1
  Mux : Mux  Inputs=3
  Mux1 : Mux  Inputs=3
  Offset : Constant  Value=1.65
  Receive1 : rtpi/Receive  Priority=12  finger_print=115482637925  blk_num=8  data_type=2
      settings: SourceProductName=Simplus Real-Time
  Receive14 : rtpi/Receive  Priority=12  finger_print=115482637925  blk_num=9  data_type=2
      settings: SourceProductName=Simplus Real-Time
  Receive2 : rtpi/Receive  Priority=12  finger_print=115482637925  blk_num=10  data_type=2
      settings: SourceProductName=Simplus Real-Time
  Receive3 : rtpi/Receive  Priority=12  finger_print=115482637925  blk_num=11  data_type=2
      settings: SourceProductName=Simplus Real-Time
  Receive4 : rtpi/Receive  Priority=12  finger_print=115482637925  blk_num=12  data_type=2
      settings: SourceProductName=Simplus Real-Time
  Receive5 : rtpi/Receive  Priority=12  finger_print=115482637925  blk_num=13  data_type=2
      settings: SourceProductName=Simplus Real-Time
  Receive6 : rtpi/Receive  Priority=12  finger_print=115482637925  blk_num=14  data_type=2
      settings: SourceProductName=Simplus Real-Time
  Voltage Divider : Gain  Gain=28.06
  Vcap : Outport
  IL : Outport  Port=2
  Vdc : Outport  Port=3
  wires:
  ADC6/1 -> Receive4/1
  Receive4/1 -> Gain/1  "Vcap1A_raw"
  Amp x INA240 x Sense Gain 6/1 -> Add6/1
  I Abs Offset 6/1 -> Add6/2
  I Abs Offset 4/1 -> Add4/2
  Amp x INA240 x Sense Gain 4/1 -> Add4/1
  ADC5/1 -> Receive2/1
  Amp x INA240 x Sense Gain 5/1 -> Add5/1
  Receive1/1 -> Gain1/1  "Vcap1B_raw"
  I Abs Offset 5/1 -> Add5/2
  Receive2/1 -> Gain2/1  "Vcap1C_raw"
  ADC4/1 -> Receive1/1
  Amp x INA240 x Sense Gain 3/1 -> Add3/1
  Amp x INA240 x Sense Gain 1/1 -> Add1/1
  I Abs Offset 1/1 -> Add1/2
  Amp x INA240 x Sense Gain 2/1 -> Add2/1
  I Abs Offset 2/1 -> Add2/2
  I Abs Offset 3/1 -> Add3/2
  Receive14/1 -> Gain3/1  "VDC1_raw"
  ADC3/1 -> Receive14/1
  Add/1 -> Voltage Divider/1
  Voltage Divider/1 -> Vdc/1  "VDC1"
  Amplifier Gain/1 -> Add/1
  Offset/1 -> Add/2
  Gain/1 -> Amp x INA240 x Sense Gain 4/1
  Gain1/1 -> Amp x INA240 x Sense Gain 5/1
  Gain2/1 -> Amp x INA240 x Sense Gain 6/1
  Gain3/1 -> Amplifier Gain/1
  Add4/1 -> Mux/1  "VcapA"
  Add5/1 -> Mux/2  "VcapB"
  Add6/1 -> Mux/3  "VcapC"
  Mux/1 -> Vcap/1
  Gain4/1 -> Amp x INA240 x Sense Gain 1/1
  Gain5/1 -> Amp x INA240 x Sense Gain 2/1
  Gain6/1 -> Amp x INA240 x Sense Gain 3/1
  Add3/1 -> Mux1/3  "VcapC"
  Mux1/1 -> Load to gen convention/1
  Add1/1 -> Mux1/1  "VcapA"
  Add2/1 -> Mux1/2  "VcapB"
  Receive3/1 -> Gain4/1  "VDC1_raw"
  ADC2/1 -> Receive3/1
  Receive5/1 -> Gain5/1  "VDC1_raw"
  ADC7/1 -> Receive5/1
  Receive6/1 -> Gain6/1  "VDC1_raw"
  ADC1/1 -> Receive6/1
  Load to gen convention/1 -> IL/1

== system Simplus_1GFM_2OFF/Voltage Controller/PI ==
  e : Inport
  RST : Inport  Port=2
  Discrete-Time Integrator : DiscreteIntegrator  gainval=1  ExternalReset=either  SampleTime=Ts  LimitOutput=on  UpperSaturationLimit=2000  LowerSaturationLimit=-2000  ICPrevOutput=DiscIntNeverNeededParam  ICPrevScaledInput=DiscIntNeverNeededParam
  Ki : Gain  Gain=Id_Integral  SaturateOnIntegerOverflow=on  OutDataTypeStr=Inherit: Same as input  ParamDataTypeStr=Inherit: Same as input
  Kp : Gain  Gain=Id_Proportional  SaturateOnIntegerOverflow=on  OutDataTypeStr=Inherit: Same as input  ParamDataTypeStr=Inherit: Same as input
  Sum4 : Sum  SaturateOnIntegerOverflow=on
  Out : Outport
  wires:
  Ki/1 -> Discrete-Time Integrator/1
  Kp/1 -> Sum4/1
  e/1 -> Ki/1, Kp/1
  Discrete-Time Integrator/1 -> Sum4/2
  Sum4/1 -> Out/1
  RST/1 -> Discrete-Time Integrator/2

== system Simplus_1GFM_2OFF/Voltage Controller/PI1 ==
  e : Inport
  RST : Inport  Port=2
  Discrete-Time Integrator : DiscreteIntegrator  gainval=1  ExternalReset=either  SampleTime=Ts  LimitOutput=on  UpperSaturationLimit=2000  LowerSaturationLimit=-2000  ICPrevOutput=DiscIntNeverNeededParam  ICPrevScaledInput=DiscIntNeverNeededParam
  Ki : Gain  Gain=Id_Integral  SaturateOnIntegerOverflow=on  OutDataTypeStr=Inherit: Same as input  ParamDataTypeStr=Inherit: Same as input
  Kp : Gain  Gain=Id_Proportional  SaturateOnIntegerOverflow=on  OutDataTypeStr=Inherit: Same as input  ParamDataTypeStr=Inherit: Same as input
  Sum4 : Sum  SaturateOnIntegerOverflow=on
  Out : Outport
  wires:
  Ki/1 -> Discrete-Time Integrator/1
  Kp/1 -> Sum4/1
  e/1 -> Ki/1, Kp/1
  Discrete-Time Integrator/1 -> Sum4/2
  Sum4/1 -> Out/1
  RST/1 -> Discrete-Time Integrator/2
